simulink model "UDP_Stateflow_LQG_FLEXOP_rbm"  (R2023a)
settings: Solver=FixedStepAuto  StartTime=0.0  StopTime=finish_time  FixedStep=input_settings.dt  RelTol=1e-3
undefined symbols (not defined in the file): controller_final, DiscIntNeverNeededParam, Discrete, f, initial_control_input, initial_control_input_SHARPy, num_cs_sharpy, num_sensors, reference_values_rbm, Rn, sys_kf, Time
libraries: slrealtimeutilitieslib x2, ctrlSharedLib x1, instrumentlib x1, slrealtimeiplib x1
settings Model: Creator=ERIK  LastModifiedBy=User
settings SolverCC: AlgebraicLoopSolver=LineSearch
settings DebuggingCC: UnconnectedInputMsg=warning  UnconnectedOutputMsg=warning  UnconnectedLineMsg=warning
settings ModelReferenceCC: EnableRefExpFcnMdlSchedulingChecks=on
settings RTWCC: DLArmComputeVersion=19.05

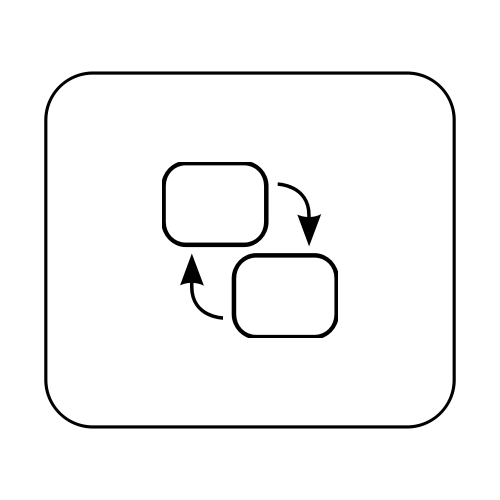
[thumbnail: Simulink's stored preview of the top-level diagram]
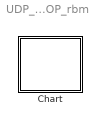
== system UDP_Stateflow_LQG_FLEXOP_rbm ==
  Chart : Stateflow chart  TreatAsAtomicUnit=on

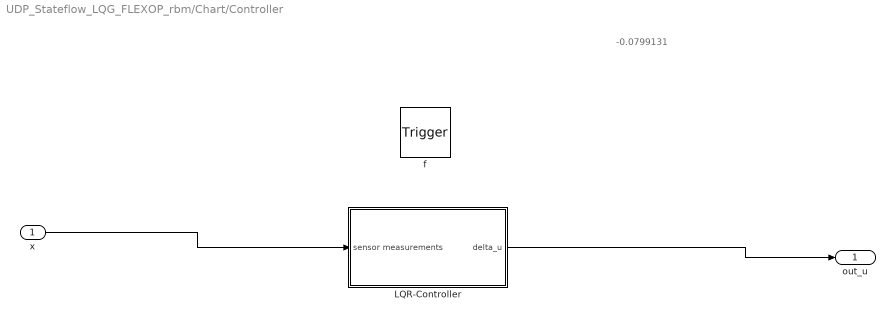
== system UDP_Stateflow_LQG_FLEXOP_rbm/Chart/Controller ==
  note: -0.0799131
  x : Inport  OutDataTypeStr=double  PortDimensions=num_sensors
  f : TriggerPort  TriggerType=function-call  VariantControl=(inherit)
      settings: CopyFcn=Stateflow.SLINSF.SimulinkMan.removeBlockPreDeleteFcn  PreDeleteFcn=Stateflow.SLINSF.SimulinkMan.unsafePredeleteFcn
  LQR-Controller : Subsystem
  out_u : Outport
  wires:
  LQR-Controller/1(delta_u) -> out_u/1
  x/1 -> LQR-Controller/1(sensor measurements)

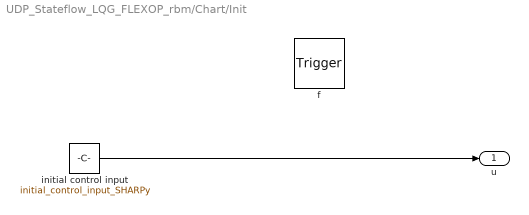
== system UDP_Stateflow_LQG_FLEXOP_rbm/Chart/Init ==
  f : TriggerPort  TriggerType=function-call  VariantControl=(inherit)
      settings: CopyFcn=Stateflow.SLINSF.SimulinkMan.removeBlockPreDeleteFcn  PreDeleteFcn=Stateflow.SLINSF.SimulinkMan.unsafePredeleteFcn
  initial control input : Constant  Value=initial_control_input_SHARPy
  u : Outport
  wires:
  initial control input/1 -> u/1

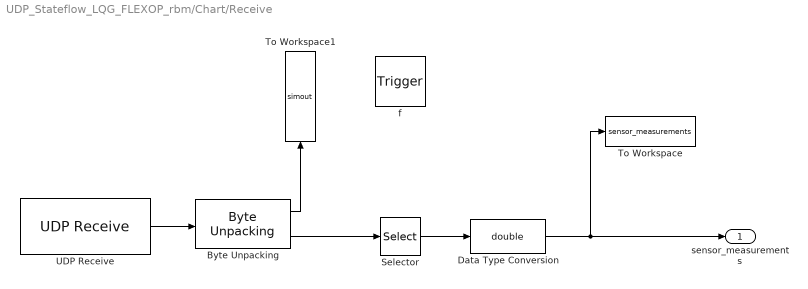
== system UDP_Stateflow_LQG_FLEXOP_rbm/Chart/Receive ==
  f : TriggerPort  TriggerType=function-call  VariantControl=(inherit)
      settings: CopyFcn=Stateflow.SLINSF.SimulinkMan.removeBlockPreDeleteFcn  PreDeleteFcn=Stateflow.SLINSF.SimulinkMan.unsafePredeleteFcn
  "Byte Unpacking " : slrealtimeutilitieslib/Byte Unpacking  MaskUnpackedDataTypes={'uint8' 'single'}  MaskUnpackedDataSizes={5 num_sensors*2}  MaskAlignment=1
  Data Type Conversion : DataTypeConversion  OutDataTypeStr=double  SaturateOnIntegerOverflow=off  RndMeth=Floor
  Selector : Selector  InputPortWidth=num_sensors*2  IndexOptions=Index vector (dialog)  Indices=2:2:2*num_sensors  OutputSizes=1
  To Workspace : ToWorkspace  VariableName=sensor_measurements  SaveFormat=Timeseries  SampleTime=-1
  To Workspace1 : ToWorkspace  VariableName=simout  SaveFormat=Timeseries  SampleTime=-1
  UDP Receive : instrumentlib/UDP Receive  LocalAddress=127.0.0.1  LocalPort=59006  EnablePortSharing=off  Host=127.0.0.1  Port=59016  GetLatestData=on  DataSize=101  DataType=uint8  ASCIIFormatting=%f,  Terminator=LF  CustomTerminator=10  ByteOrder=little-endian  EnableBlockingMode=on  Timeout=600  SampleTime=-1  SimulateUsing=Interpreted execution
  sensor_measurements : Outport
  wires:
  UDP Receive/1 -> "Byte Unpacking "/1
  Selector/1 -> Data Type Conversion/1
  Data Type Conversion/1 -> To Workspace/1, sensor_measurements/1
  "Byte Unpacking "/2 -> Selector/1
  "Byte Unpacking "/1 -> To Workspace1/1

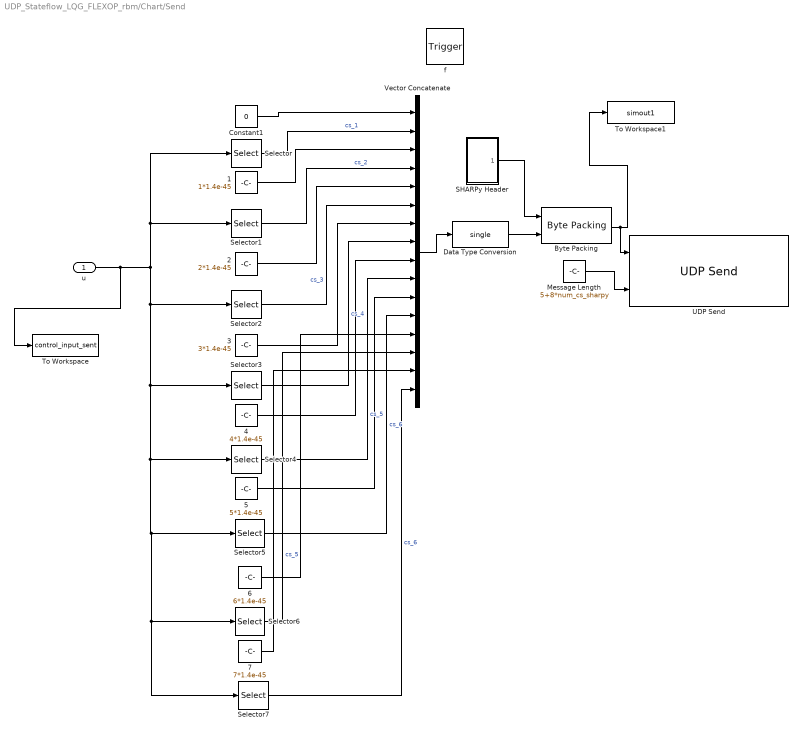
== system UDP_Stateflow_LQG_FLEXOP_rbm/Chart/Send ==
  u : Inport  OutDataTypeStr=double  PortDimensions=num_cs_sharpy
  f : TriggerPort  TriggerType=function-call  VariantControl=(inherit)
      settings: CopyFcn=Stateflow.SLINSF.SimulinkMan.removeBlockPreDeleteFcn  PreDeleteFcn=Stateflow.SLINSF.SimulinkMan.unsafePredeleteFcn
  1 : Constant  Value=1*1.4e-45
  2 : Constant  Value=2*1.4e-45
  3 : Constant  Value=3*1.4e-45
  4 : Constant  Value=4*1.4e-45
  5 : Constant  Value=5*1.4e-45
  6 : Constant  Value=6*1.4e-45
  7 : Constant  Value=7*1.4e-45
  "Byte Packing " : slrealtimeutilitieslib/Byte Packing  MaskPackedDataType=uint8  MaskUnpackedDataTypes={'uint8' 'single'}  MaskAlignment=1
  Constant1 : Constant  Value=0
  Data Type Conversion : DataTypeConversion  OutDataTypeStr=single  SaturateOnIntegerOverflow=off  RndMeth=Floor
  Message Length : Constant  Value=5+8*num_cs_sharpy
  SHARPy Header : Subsystem
  Selector : Selector  InputPortWidth=num_cs_sharpy  IndexOptions=Index vector (dialog)  Indices=[1]  OutputSizes=1
  Selector1 : Selector  InputPortWidth=num_cs_sharpy  IndexOptions=Index vector (dialog)  Indices=[2]  OutputSizes=1
  Selector2 : Selector  InputPortWidth=num_cs_sharpy  IndexOptions=Index vector (dialog)  Indices=[3]  OutputSizes=1
  Selector3 : Selector  InputPortWidth=num_cs_sharpy  IndexOptions=Index vector (dialog)  Indices=[4]  OutputSizes=1
  Selector4 : Selector  InputPortWidth=num_cs_sharpy  IndexOptions=Index vector (dialog)  Indices=[5]  OutputSizes=1
  Selector5 : Selector  InputPortWidth=num_cs_sharpy  IndexOptions=Index vector (dialog)  Indices=[6]  OutputSizes=1
  Selector6 : Selector  InputPortWidth=num_cs_sharpy  IndexOptions=Index vector (dialog)  Indices=[7]  OutputSizes=1
  Selector7 : Selector  InputPortWidth=num_cs_sharpy  IndexOptions=Index vector (dialog)  Indices=[8]  OutputSizes=1
  To Workspace : ToWorkspace  VariableName=control_input_sent  SaveFormat=Timeseries  SampleTime=-1
  To Workspace1 : ToWorkspace  VariableName=simout1  SaveFormat=Timeseries  SampleTime=-1
  UDP Send : slrealtimeiplib/UDP Send  useHostTargetConn=on  toAddress=127.0.0.1  toPort=64016  sampleTime=-1  enableMessage=off  localPort=59001
  Vector Concatenate : Concatenate  NumInputs=16
  wires:
  u/1 -> To Workspace/1, Selector/1, Selector1/1, Selector7/1, Selector6/1, Selector5/1, Selector4/1, Selector3/1, Selector2/1
  Selector/1 -> Vector Concatenate/2  "cs_1"
  Constant1/1 -> Vector Concatenate/1
  Data Type Conversion/1 -> "Byte Packing "/2
  "Byte Packing "/1 -> To Workspace1/1, UDP Send/1
  Message Length/1 -> UDP Send/2
  SHARPy Header/1(Header) -> "Byte Packing "/1
  Selector1/1 -> Vector Concatenate/4  "cs_2"
  Selector2/1 -> Vector Concatenate/6  "cs_3"
  Selector3/1 -> Vector Concatenate/8  "cs_4"
  1/1 -> Vector Concatenate/3
  2/1 -> Vector Concatenate/5
  3/1 -> Vector Concatenate/7
  Vector Concatenate/1 -> Data Type Conversion/1
  4/1 -> Vector Concatenate/9
  Selector4/1 -> Vector Concatenate/10  "cs_5"
  5/1 -> Vector Concatenate/11
  Selector5/1 -> Vector Concatenate/12  "cs_6"
  6/1 -> Vector Concatenate/13
  Selector6/1 -> Vector Concatenate/14  "cs_5"
  7/1 -> Vector Concatenate/15
  Selector7/1 -> Vector Concatenate/16  "cs_6"

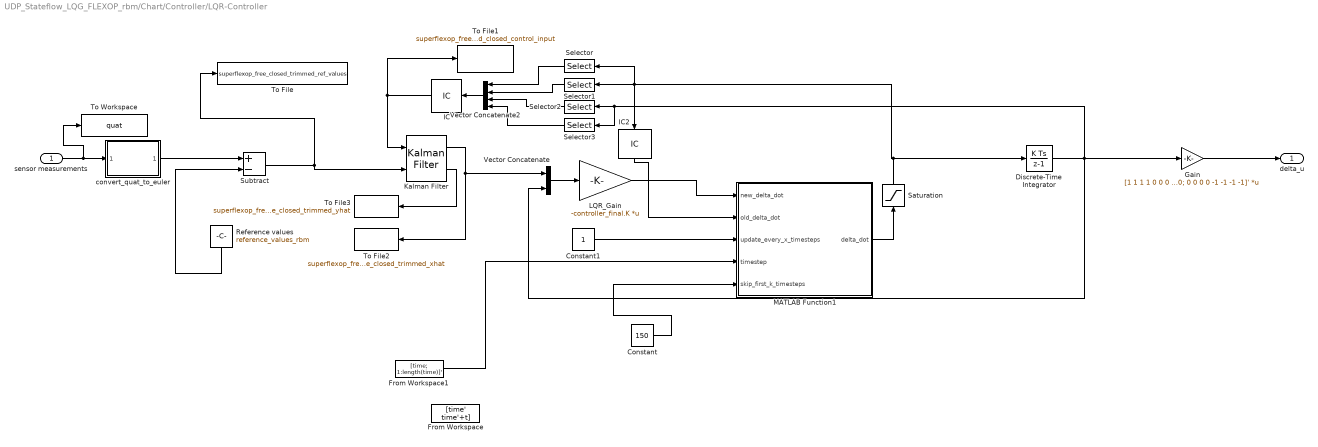
== system UDP_Stateflow_LQG_FLEXOP_rbm/Chart/Controller/LQR-Controller ==
  sensor measurements : Inport
  Constant : Constant  Value=150
  Constant1 : Constant
  Discrete-Time Integrator : DiscreteIntegrator  SampleTime=-1  ICPrevOutput=DiscIntNeverNeededParam  ICPrevScaledInput=DiscIntNeverNeededParam
  From Workspace : FromWorkspace  VariableName=[time' time'+t]  SampleTime=-1
  From Workspace1 : FromWorkspace  VariableName=[time; 1:length(time)]'  SampleTime=-1
  Gain : Gain  Gain=[1 1 1 1 0 0 0 0; 0 0 0 0 -1 -1 -1 -1]'  Multiplication=Matrix(K*u)
  IC : InitialCondition  Value=initial_control_input
  IC2 : InitialCondition  Value=0
  Kalman Filter : ctrlSharedLib/Kalman Filter  TimeDomain=Discrete-Time  UseCurrentEstimator=on  ModelSource=Individual A, B, C, D matrices  ModelSourceVariable=ss(0.95,1,1,0,1)  A=sys_kf.A  B=sys_kf.B(:,1:end-1)  C=sys_kf.C  D=sys_kf.D(:,1:end-1)  NumberOfStates=1  NumberOfInputs=1  NumberOfOutputs=1  InitialEstimateSource=Dialog  X0=0  P0=10  UseK=off  UseGH=on  NumberOfProcessNoiseInputs=1  G=sys_kf.B(:,end)  TimeInvariantG=on  H=sys_kf.D(:,end)  TimeInvariantH=on  Q=Qn  TimeInvariantQ=on  R=Rn  TimeInvariantR=on  N=0  TimeInvariantN=on  AddInputPort=on  AddEnablePort=off  OutputEstimatedY=on  OutputP=off  Ts=-1
  LQR_Gain : Gain  Gain=-controller_final.K  Multiplication=Matrix(K*u) (u vector)
  MATLAB Function1 : MATLAB Function  TreatAsAtomicUnit=on
  Reference values : Constant  Value=reference_values_rbm
  Saturation : Saturate  UpperLimit=deg2rad(50)  LowerLimit=-deg2rad(50)
  Selector : Selector  InputPortWidth=num_cs  IndexOptions=Index vector (dialog)  Indices=[1]  OutputSizes=1
  Selector1 : Selector  InputPortWidth=2  IndexOptions=Index vector (dialog)  Indices=[2]  OutputSizes=1
  Selector2 : Selector  InputPortWidth=num_cs  IndexOptions=Index vector (dialog)  Indices=[1]  OutputSizes=1
  Selector3 : Selector  InputPortWidth=2  IndexOptions=Index vector (dialog)  Indices=[2]  OutputSizes=1
  Subtract : Sum  Inputs=+-
  To File : ToFile  Filename=superflexop_free_closed_trimmed_ref_values  MatrixName=reference_value_correction  SaveFormat=Timeseries
  To File1 : ToFile  Filename=superflexop_free_trimmed_closed_control_input  MatrixName=known_input_kalman  SaveFormat=Timeseries
  To File2 : ToFile  Filename=superflexop_free_closed_trimmed_xhat  MatrixName=xhat  SaveFormat=Timeseries
  To File3 : ToFile  Filename=superflexop_free_closed_trimmed_yhat  MatrixName=yhat  SaveFormat=Timeseries
  To Workspace : ToWorkspace  VariableName=quat  SaveFormat=Timeseries  SampleTime=-1
  Vector Concatenate : Concatenate
  Vector Concatenate2 : Concatenate  NumInputs=4
  convert_quat_to_euler : MATLAB Function  TreatAsAtomicUnit=on
  delta_u : Outport
  wires:
  Vector Concatenate/1 -> LQR_Gain/1
  Vector Concatenate2/1 -> IC/1
  Discrete-Time Integrator/1 -> Selector3/1, Selector2/1, Vector Concatenate/2, Gain/1
  Gain/1 -> delta_u/1
  Reference values/1 -> Subtract/2
  Subtract/1 -> To File/1, Kalman Filter/2
  IC/1 -> Kalman Filter/1, To File1/1
  LQR_Gain/1 -> MATLAB Function1/1(new_delta_dot)
  Kalman Filter/2 -> To File3/1
  Kalman Filter/1 -> To File2/1, Vector Concatenate/1
  MATLAB Function1/1(delta_dot) -> Saturation/1
  Constant1/1 -> MATLAB Function1/3(update_every_x_timesteps)
  IC2/1 -> MATLAB Function1/2(old_delta_dot)
  From Workspace1/1 -> MATLAB Function1/4(timestep)
  Constant/1 -> MATLAB Function1/5(skip_first_k_timesteps)
  Saturation/1 -> IC2/1, Selector1/1, Selector/1, Discrete-Time Integrator/1
  sensor measurements/1 -> To Workspace/1, convert_quat_to_euler/1(sensor_measurements)
  convert_quat_to_euler/1(sensor_measurements_incl_euler) -> Subtract/1
  Selector/1 -> Vector Concatenate2/1
  Selector1/1 -> Vector Concatenate2/2
  Selector2/1 -> Vector Concatenate2/3
  Selector3/1 -> Vector Concatenate2/4

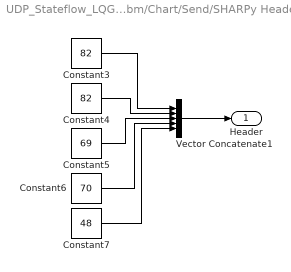
== system UDP_Stateflow_LQG_FLEXOP_rbm/Chart/Send/SHARPy Header ==
  Constant3 : Constant  Value=82  OutDataTypeStr=uint8
  Constant4 : Constant  Value=82  OutDataTypeStr=uint8
  Constant5 : Constant  Value=69  OutDataTypeStr=uint8
  Constant6 : Constant  Value=70  OutDataTypeStr=uint8
  Constant7 : Constant  Value=48  OutDataTypeStr=uint8
  Vector Concatenate1 : Concatenate  NumInputs=5
  Header : Outport
  wires:
  Constant7/1 -> Vector Concatenate1/5
  Constant5/1 -> Vector Concatenate1/3
  Constant6/1 -> Vector Concatenate1/4
  Constant4/1 -> Vector Concatenate1/2
  Constant3/1 -> Vector Concatenate1/1
  Vector Concatenate1/1 -> Header/1

== matlab function UDP_Stateflow_LQG_FLEXOP_rbm/Chart/Controller/LQR-Controller/MATLAB Function1 ==
  data: delta_dot output; new_delta_dot input; old_delta_dot input; update_every_x_timesteps input; timestep input; skip_first_k_timesteps input
function delta_dot = enforce_controller_bandwith(new_delta_dot, old_delta_dot, update_every_x_timesteps, timestep, skip_first_k_timesteps)

if timestep > skip_first_k_timesteps

    r = mod(timestep, update_every_x_timesteps);
    if r == 0
        delta_dot = new_delta_dot;
    else
        delta_dot = old_delta_dot;
    end
else
    delta_dot = old_delta_dot;
end
% delta_dot = squeeze(delta_dot)
end

== matlab function UDP_Stateflow_LQG_FLEXOP_rbm/Chart/Controller/LQR-Controller/convert_quat_to_euler ==
  data: sensor_measurements input; sensor_measurements_incl_euler output
function sensor_measurements_incl_euler = fcn(sensor_measurements)
    %%   Transform Quaternion in measurements to Euler angles.
    
    quat = sensor_measurements(end-3:end)'    
    euler = quat2eul(quat);
    sensor_measurements_incl_euler = [sensor_measurements(1:end-4)' euler];
end

== stateflow chart UDP_Stateflow_LQG_FLEXOP_rbm/Chart ==
  state u=Init [function]
  state Send(u) [function]
  state Stateflow
    entry:  u=Init();
    during: Send(u);
    x =Receive();
    u = Controller(x);
  state sensor_measurements = Receive [function]
  state out_u = Controller(x) [function]
  (default) -> Stateflow
  data: u function_output; u function_input double size=num_cs_sharpy; sensor_measurements function_output; out_u function_output; x function_input double size=num_sensors; x local; u local
